simulink model "sldemo_absbrake_ATESST2008b"  (Simulink 7.2)
settings: Solver=ode45  StartTime=0.0  StopTime=10.0  RelTol=1e-3
settings Model: Creator=carlj  LastModifiedBy=carlj

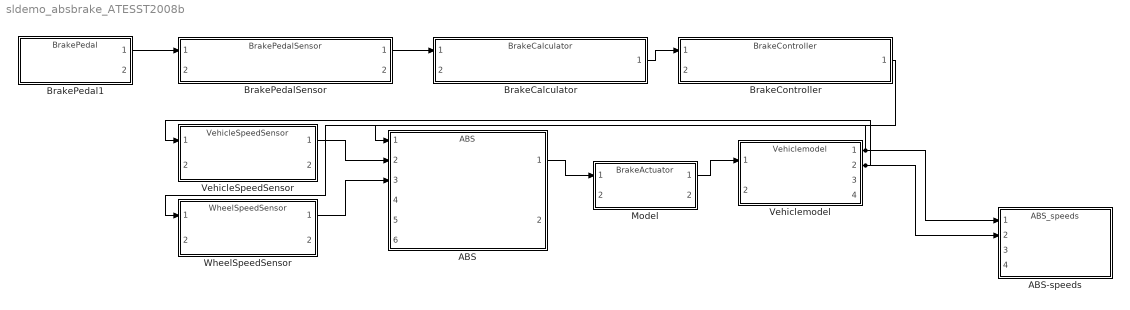
== system sldemo_absbrake_ATESST2008b ==
  ABS : ModelReference  ModelName=ABS  SimulationMode=Accelerator  ModelReferenceVersion=1.18  CopyOfModelName=ABS
  ABS-speeds : ModelReference  ModelName=ABS_speeds  SimulationMode=Accelerator  ModelReferenceVersion=1.14  CopyOfModelName=ABS_speeds
  BrakeCalculator : ModelReference  ModelName=BrakeCalculator  SimulationMode=Accelerator  ModelReferenceVersion=1.17  CopyOfModelName=BrakeCalculator
  BrakeController : ModelReference  ModelName=BrakeController  SimulationMode=Accelerator  ModelReferenceVersion=1.17  CopyOfModelName=BrakeController
  BrakePedal1 : ModelReference  ModelName=BrakePedal  SimulationMode=Accelerator  ModelReferenceVersion=1.16  CopyOfModelName=BrakePedal
  BrakePedalSensor : ModelReference  ModelName=BrakePedalSensor  SimulationMode=Accelerator  ModelReferenceVersion=1.18  CopyOfModelName=BrakePedalSensor
  Model : ModelReference  ModelName=BrakeActuator  SimulationMode=Accelerator  ModelReferenceVersion=1.3  CopyOfModelName=BrakeActuator
  VehicleSpeedSensor : ModelReference  ModelName=VehicleSpeedSensor  SimulationMode=Accelerator  ModelReferenceVersion=1.19  CopyOfModelName=VehicleSpeedSensor
  Vehiclemodel : ModelReference  ModelName=Vehiclemodel  SimulationMode=Accelerator  ModelReferenceVersion=1.19  CopyOfModelName=Vehiclemodel
  "WheelSpeedSensor " : ModelReference  ModelName=WheelSpeedSensor  SimulationMode=Accelerator  ModelReferenceVersion=1.19  CopyOfModelName=WheelSpeedSensor
  wires:
  BrakeController/1 -> ABS/1
  VehicleSpeedSensor/1 -> ABS/2
  "WheelSpeedSensor "/1 -> ABS/3
  ABS/1 -> Model/1
  Vehiclemodel/1 -> ABS-speeds/1, "WheelSpeedSensor "/1
  Vehiclemodel/2 -> ABS-speeds/2, VehicleSpeedSensor/1
  BrakePedalSensor/1 -> BrakeCalculator/1
  BrakeCalculator/1 -> BrakeController/1
  BrakePedal1/1 -> BrakePedalSensor/1
  Model/1 -> Vehiclemodel/1
